simulink model "adrc_controller"  (R2020a)
settings: Solver=ode45  StartTime=0.0  StopTime=5  FixedStep=1e-4  RelTol=1e-4  EnableMultiTasking=on
values from neighbouring files (symbols this model uses):
  b0 = 0.83    [eso.m]
undefined symbols (not defined in the file or in its folder): kd, kp
settings Model: Creator=kbmaj  LastModifiedBy=MIWAN
settings DataIOCC: LimitDataPoints=on  SaveFormat=Array  ReturnWorkspaceOutputs=off
settings OptimizationCC: LifeSpan=inf
settings DebuggingCC: SFUnexpectedBacktrackingDiag=warning  SFNoUnconditionalDefaultTransitionDiag=warning  SFExecutionAtInitializationDiag=none  ArithmeticOperatorsInVariantConditions=warning
settings HardwareCC: ProdBitPerPointer=32  ProdBitPerSizeT=32  ProdBitPerPtrDiffT=32  ProdLargestAtomicFloat=None  ProdIntDivRoundTo=Undefined  ProdEndianess=Unspecified  ProdWordSize=32  ProdHWDeviceType=32-bit Generic
settings ModelReferenceCC: PropagateSignalLabelsOutOfModel=off
settings SFSimCC: SimUseLocalCustomCode=off  CustomCodeUndefinedFunction=UseInterfaceOnly
settings RTWCC: RTWUseLocalCustomCode=off
settings CodeAppCC: StateflowObjectComments=on
settings GRTTargetCC: TargetLangStandard=C89/C90 (ANSI)
settings ConfigComp: CovMetricSettings=dw  CovHtmlReporting=on  CovSaveCumulativeToWorkspaceVar=on  CovSaveSingleToWorkspaceVar=on  CovExternalEMLEnable=off

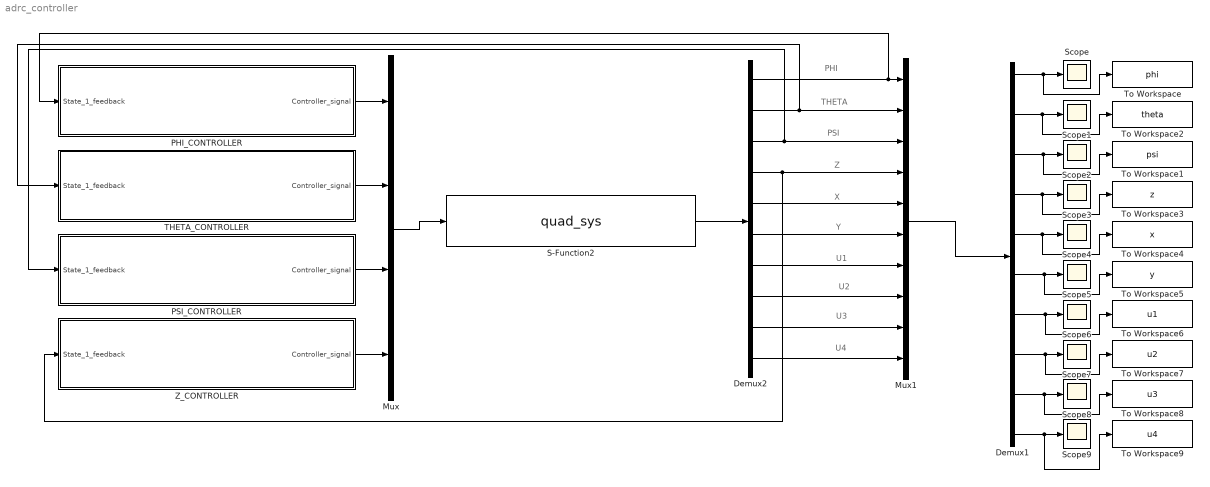
== system adrc_controller ==
  note: U4
  note: U3
  note: U2
  note: U1
  note: Y
  note: X
  note: Z
  note: PSI
  note: THETA
  note: PHI
  Demux1 : Demux  Outputs=10
  Demux2 : Demux  Outputs=10
  Mux : Mux
  Mux1 : Mux  Inputs=10
  PHI_CONTROLLER : Subsystem
  PSI_CONTROLLER : Subsystem
  S-Function2 : S-Function  FunctionName=quad_sys  SFunctionDeploymentMode=off  EnableBusSupport=off
  Scope{,1..9} (10 alike) : Scope
  THETA_CONTROLLER : Subsystem
  To Workspace : ToWorkspace  VariableName=phi  SaveFormat=Timeseries  SampleTime=-1
  To Workspace1 : ToWorkspace  VariableName=psi  SaveFormat=Timeseries  SampleTime=-1
  To Workspace2 : ToWorkspace  VariableName=theta  SaveFormat=Timeseries  SampleTime=-1
  To Workspace3 : ToWorkspace  VariableName=z  SaveFormat=Timeseries  SampleTime=-1
  To Workspace4 : ToWorkspace  VariableName=x  SaveFormat=Timeseries  SampleTime=-1
  To Workspace5 : ToWorkspace  VariableName=y  SaveFormat=Timeseries  SampleTime=-1
  To Workspace6 : ToWorkspace  VariableName=u1  SaveFormat=Timeseries  SampleTime=-1
  To Workspace7 : ToWorkspace  VariableName=u2  SaveFormat=Timeseries  SampleTime=-1
  To Workspace8 : ToWorkspace  VariableName=u3  SaveFormat=Timeseries  SampleTime=-1
  To Workspace9 : ToWorkspace  VariableName=u4  SaveFormat=Timeseries  SampleTime=-1
  Z_CONTROLLER : Subsystem
  wires:
  S-Function2/1 -> Demux2/1
  Mux/1 -> S-Function2/1
  PHI_CONTROLLER/1(Controller_signal) -> Mux/1
  Demux2/10 -> Mux1/10
  Demux2/9 -> Mux1/9
  Demux2/8 -> Mux1/8
  Demux2/7 -> Mux1/7
  Demux2/6 -> Mux1/6
  Demux2/5 -> Mux1/5
  Demux2/4 -> Z_CONTROLLER/1(State_1_feedback), Mux1/4
  Demux2/3 -> PSI_CONTROLLER/1(State_1_feedback), Mux1/3
  Demux2/2 -> THETA_CONTROLLER/1(State_1_feedback), Mux1/2
  Demux2/1 -> PHI_CONTROLLER/1(State_1_feedback), Mux1/1
  Mux1/1 -> Demux1/1
  Demux1/1 -> To Workspace/1, Scope/1
  Demux1/2 -> Scope1/1, To Workspace2/1
  Demux1/3 -> Scope2/1, To Workspace1/1
  Demux1/4 -> To Workspace3/1, Scope3/1
  Demux1/5 -> To Workspace4/1, Scope4/1
  Demux1/6 -> To Workspace5/1, Scope5/1
  Demux1/7 -> To Workspace6/1, Scope6/1
  Demux1/8 -> To Workspace7/1, Scope7/1
  Demux1/9 -> To Workspace8/1, Scope8/1
  Demux1/10 -> To Workspace9/1, Scope9/1
  PSI_CONTROLLER/1(Controller_signal) -> Mux/3
  THETA_CONTROLLER/1(Controller_signal) -> Mux/2
  Z_CONTROLLER/1(Controller_signal) -> Mux/4

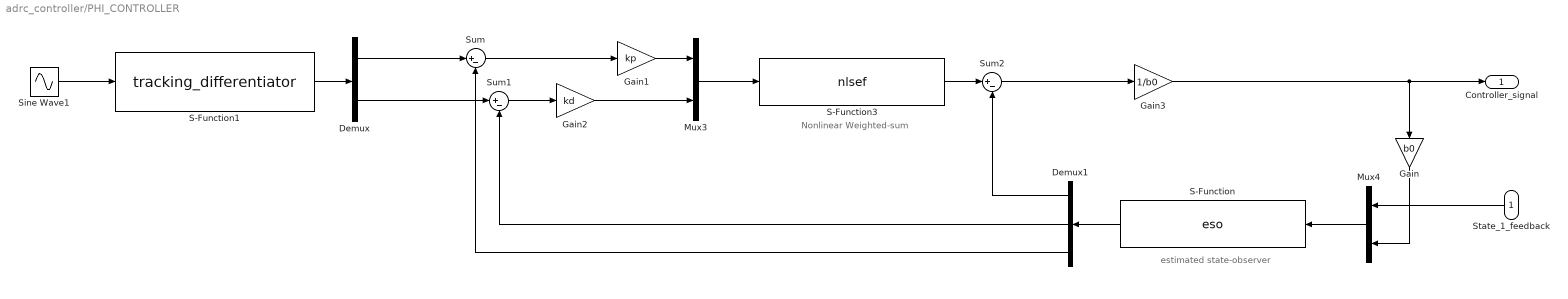
== system adrc_controller/PHI_CONTROLLER ==
  note: estimated state-observer
  note: Nonlinear Weighted-sum
  State_1_feedback : Inport
  Demux : Demux  Outputs=2
  Demux1 : Demux  Outputs=3
  Gain : Gain  Gain=b0
  Gain1 : Gain  Gain=kp
  Gain2 : Gain  Gain=kd
  Gain3 : Gain  Gain=1/b0
  Mux3 : Mux  Inputs=2
  Mux4 : Mux  Inputs=2
  S-Function : S-Function  FunctionName=eso  SFunctionDeploymentMode=off  EnableBusSupport=off
  S-Function1 : S-Function  FunctionName=tracking_differentiator  SFunctionDeploymentMode=off  EnableBusSupport=off
  S-Function3 : S-Function  FunctionName=nlsef  SFunctionDeploymentMode=off  EnableBusSupport=off
  Sine Wave1 : Sin  SampleTime=0
  Sum : Sum  Inputs=|+-
  Sum1 : Sum  Inputs=|+-
  Sum2 : Sum  Inputs=|+-
  Controller_signal : Outport
  wires:
  Mux3/1 -> S-Function3/1
  Mux4/1 -> S-Function/1
  S-Function/1 -> Demux1/1
  Sum/1 -> Gain1/1
  Demux/1 -> Sum/1
  Demux/2 -> Sum1/1
  Sum1/1 -> Gain2/1
  Gain1/1 -> Mux3/1
  Gain2/1 -> Mux3/2
  S-Function3/1 -> Sum2/1
  Sum2/1 -> Gain3/1
  Gain3/1 -> Controller_signal/1, Gain/1
  Demux1/1 -> Sum2/2
  Demux1/3 -> Sum/2
  Demux1/2 -> Sum1/2
  Gain/1 -> Mux4/2
  State_1_feedback/1 -> Mux4/1
  Sine Wave1/1 -> S-Function1/1
  S-Function1/1 -> Demux/1

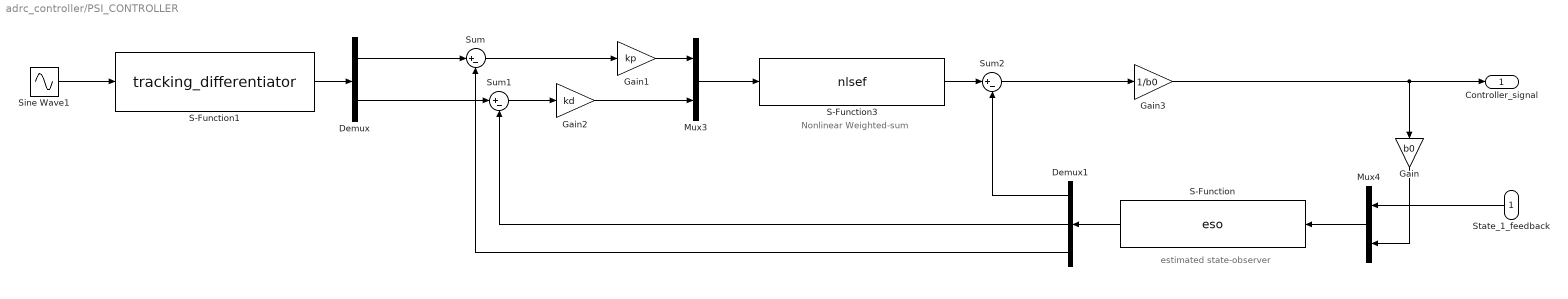
== system adrc_controller/PSI_CONTROLLER ==
  note: estimated state-observer
  note: Nonlinear Weighted-sum
  State_1_feedback : Inport
  Demux : Demux  Outputs=2
  Demux1 : Demux  Outputs=3
  Gain : Gain  Gain=b0
  Gain1 : Gain  Gain=kp
  Gain2 : Gain  Gain=kd
  Gain3 : Gain  Gain=1/b0
  Mux3 : Mux  Inputs=2
  Mux4 : Mux  Inputs=2
  S-Function : S-Function  FunctionName=eso  SFunctionDeploymentMode=off  EnableBusSupport=off
  S-Function1 : S-Function  FunctionName=tracking_differentiator  SFunctionDeploymentMode=off  EnableBusSupport=off
  S-Function3 : S-Function  FunctionName=nlsef  SFunctionDeploymentMode=off  EnableBusSupport=off
  Sine Wave1 : Sin  SampleTime=0
  Sum : Sum  Inputs=|+-
  Sum1 : Sum  Inputs=|+-
  Sum2 : Sum  Inputs=|+-
  Controller_signal : Outport
  wires:
  Sine Wave1/1 -> S-Function1/1
  Sum/1 -> Gain1/1
  State_1_feedback/1 -> Mux4/1
  Gain1/1 -> Mux3/1
  Sum2/1 -> Gain3/1
  Demux1/3 -> Sum/2
  Gain3/1 -> Controller_signal/1, Gain/1
  Mux4/1 -> S-Function/1
  Mux3/1 -> S-Function3/1
  S-Function/1 -> Demux1/1
  Demux/1 -> Sum/1
  S-Function3/1 -> Sum2/1
  S-Function1/1 -> Demux/1
  Demux1/1 -> Sum2/2
  Gain2/1 -> Mux3/2
  Demux/2 -> Sum1/1
  Sum1/1 -> Gain2/1
  Gain/1 -> Mux4/2
  Demux1/2 -> Sum1/2

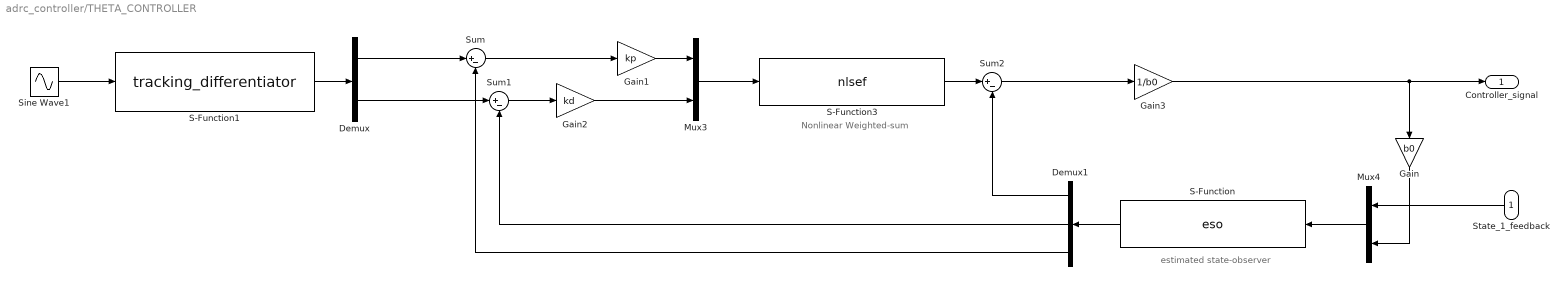
== system adrc_controller/THETA_CONTROLLER ==
  note: estimated state-observer
  note: Nonlinear Weighted-sum
  State_1_feedback : Inport
  Demux : Demux  Outputs=2
  Demux1 : Demux  Outputs=3
  Gain : Gain  Gain=b0
  Gain1 : Gain  Gain=kp
  Gain2 : Gain  Gain=kd
  Gain3 : Gain  Gain=1/b0
  Mux3 : Mux  Inputs=2
  Mux4 : Mux  Inputs=2
  S-Function : S-Function  FunctionName=eso  SFunctionDeploymentMode=off  EnableBusSupport=off
  S-Function1 : S-Function  FunctionName=tracking_differentiator  SFunctionDeploymentMode=off  EnableBusSupport=off
  S-Function3 : S-Function  FunctionName=nlsef  SFunctionDeploymentMode=off  EnableBusSupport=off
  Sine Wave1 : Sin  SampleTime=0
  Sum : Sum  Inputs=|+-
  Sum1 : Sum  Inputs=|+-
  Sum2 : Sum  Inputs=|+-
  Controller_signal : Outport
  wires:
  Sine Wave1/1 -> S-Function1/1
  Sum/1 -> Gain1/1
  State_1_feedback/1 -> Mux4/1
  Gain1/1 -> Mux3/1
  Sum2/1 -> Gain3/1
  Demux1/3 -> Sum/2
  Gain3/1 -> Controller_signal/1, Gain/1
  Mux4/1 -> S-Function/1
  Mux3/1 -> S-Function3/1
  S-Function/1 -> Demux1/1
  Demux/1 -> Sum/1
  S-Function3/1 -> Sum2/1
  S-Function1/1 -> Demux/1
  Demux1/1 -> Sum2/2
  Gain2/1 -> Mux3/2
  Demux/2 -> Sum1/1
  Sum1/1 -> Gain2/1
  Gain/1 -> Mux4/2
  Demux1/2 -> Sum1/2

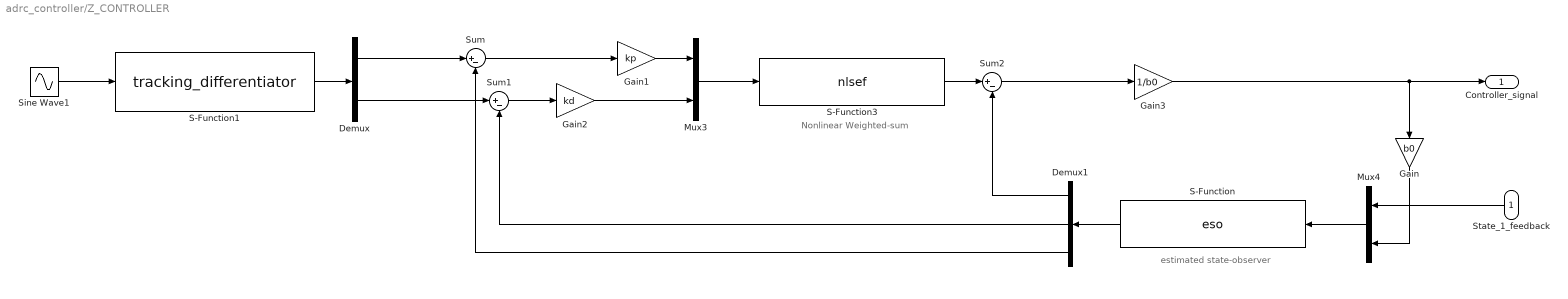
== system adrc_controller/Z_CONTROLLER ==
  note: estimated state-observer
  note: Nonlinear Weighted-sum
  State_1_feedback : Inport
  Demux : Demux  Outputs=2
  Demux1 : Demux  Outputs=3
  Gain : Gain  Gain=b0
  Gain1 : Gain  Gain=kp
  Gain2 : Gain  Gain=kd
  Gain3 : Gain  Gain=1/b0
  Mux3 : Mux  Inputs=2
  Mux4 : Mux  Inputs=2
  S-Function : S-Function  FunctionName=eso  SFunctionDeploymentMode=off  EnableBusSupport=off
  S-Function1 : S-Function  FunctionName=tracking_differentiator  SFunctionDeploymentMode=off  EnableBusSupport=off
  S-Function3 : S-Function  FunctionName=nlsef  SFunctionDeploymentMode=off  EnableBusSupport=off
  Sine Wave1 : Sin  SampleTime=0
  Sum : Sum  Inputs=|+-
  Sum1 : Sum  Inputs=|+-
  Sum2 : Sum  Inputs=|+-
  Controller_signal : Outport
  wires:
  Sine Wave1/1 -> S-Function1/1
  Sum/1 -> Gain1/1
  State_1_feedback/1 -> Mux4/1
  Gain1/1 -> Mux3/1
  Sum2/1 -> Gain3/1
  Demux1/3 -> Sum/2
  Gain3/1 -> Controller_signal/1, Gain/1
  Mux4/1 -> S-Function/1
  Mux3/1 -> S-Function3/1
  S-Function/1 -> Demux1/1
  Demux/1 -> Sum/1
  S-Function3/1 -> Sum2/1
  S-Function1/1 -> Demux/1
  Demux1/1 -> Sum2/2
  Gain2/1 -> Mux3/2
  Demux/2 -> Sum1/1
  Sum1/1 -> Gain2/1
  Gain/1 -> Mux4/2
  Demux1/2 -> Sum1/2
